simulink model "FFT_Module4"  (R2021a)
settings: Solver=VariableStepAuto  StartTime=0.0  StopTime=10  RelTol=1e-3
libraries: dspxfrm3 x1
settings Model: Creator=ujjai  LastModifiedBy=ujjai

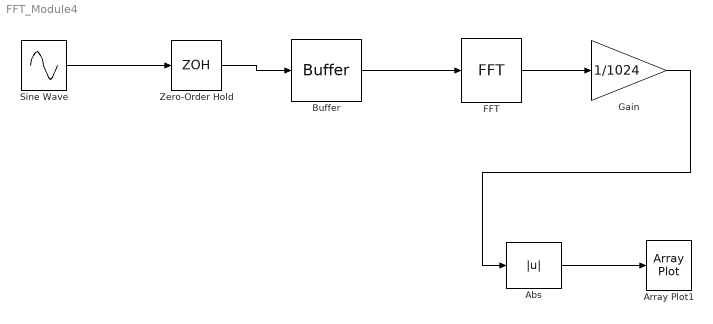
== system FFT_Module4 ==
  Abs : Abs
  Array Plot1 : ArrayPlot  WindowPosition=[1.000000,41.000000,1707.000000,1004.000000,]  YLimits=[0.001,569.5567195789555]  DefaultConfigurationName=dsp.scopes.ArrayPlotBlockSpecification
  Buffer : Buffer  N=1024  OutputFrames=off
  FFT : dspxfrm3/FFT  FFTImplementation=Auto  CompMethod=Table lookup  TableOpt=NEW  TableOptActive=Speed  BitRevOrder=off  Normalize=off  InheritFFTLength=off  FFTLength=4096  WrapInput=off  roundingMode=Floor  overflowMode=off  firstCoeffDataTypeStr=Inherit: Same word length as input  firstCoeffLastDataTypeStr=Inherit: Same word length as input  outputMin=[]  outputMax=[]
  Gain : Gain  Gain=1/1024
  Sine Wave : Sin  Frequency=6308.3180412  SampleTime=0
  Zero-Order Hold : ZeroOrderHold  SampleTime=1e-5
  wires:
  Sine Wave/1 -> Zero-Order Hold/1
  Zero-Order Hold/1 -> Buffer/1
  Buffer/1 -> FFT/1
  FFT/1 -> Gain/1
  Gain/1 -> Abs/1
  Abs/1 -> Array Plot1/1
